simulink model "prob_8"  (R2020b)
settings: Solver=VariableStepAuto  StartTime=0.0  StopTime=10.0  RelTol=1e-3
settings Model: Creator=Akshay A H  LastModifiedBy=Akshay A H

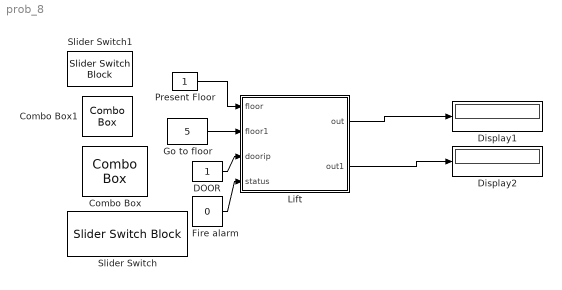
== system prob_8 ==
  Combo Box : ComboBox  SelectedLabel=FLOOR4
      settings: Values={{'GROUND', 'FLOOR1', 'FLOOR2', 'FLOOR3', 'FLOOR4'}, [1 2 3 4 5]}
  Combo Box1 : ComboBox  SelectedLabel=GROUND
      settings: Values={{'GROUND', 'FLOOR1', 'FLOOR2', 'FLOOR3', 'FLOOR4'}, [1 2 3 4 5]}
  DOOR : Constant
  Display1 : Display
  Display2 : Display
  Fire alarm : Constant  Value=0
  Go to floor : Constant  Value=5
  Lift : Stateflow chart  TreatAsAtomicUnit=on
  Present Floor : Constant
  Slider Switch : SliderSwitchBlock
      settings: Values={{'Off', 'On'}, [0 1]}
  Slider Switch1 : SliderSwitchBlock
      settings: Values={{'Off', 'On'}, [0 1]}
  wires:
  Present Floor/1 -> Lift/1(floor)
  Lift/1(out) -> Display1/1
  Lift/2(out1) -> Display2/1
  DOOR/1 -> Lift/3(doorip)
  Go to floor/1 -> Lift/2(floor1)
  Fire alarm/1 -> Lift/4(status)

== stateflow chart prob_8/Lift ==
  state Start
    (history)
    state Lift_For_five_floor
      (history)
      state Floor1
        entry:
        present=1;
        out=1;
      state Floor2
        entry:
        out=2;
        present=out;
      state Floor3
        entry:
        out=3;
        present=out;
      state Floor4
        entry:
        out=4;
        present=out;
      state Floor5
        entry:
        out=5;
        present=out
      Start.Lift_For_five_floor.Floor1 -> Start.Lift_For_five_floor.Floor1 [order 2] : [present==floor]
      (default) -> Start.Lift_For_five_floor.Floor1
      Start.Lift_For_five_floor.Floor3 -> Start.Lift_For_five_floor.Floor4 [order 1] : [present<floor]
      Start.Lift_For_five_floor.Floor2 -> Start.Lift_For_five_floor.Floor3 [order 1] : [present<floor]
      Start.Lift_For_five_floor.Floor4 -> Start.Lift_For_five_floor.Floor5 [order 1] : [present<floor]
      Start.Lift_For_five_floor.Floor1 -> Start.Lift_For_five_floor.Floor2 [order 1] : [present<floor]
      Start.Lift_For_five_floor.Floor5 -> Start.Lift_For_five_floor.Floor5 [order 2] : [floor==present]
      Start.Lift_For_five_floor.Floor5 -> Start.Lift_For_five_floor.Floor4 [order 1] : [present>floor]
      Start.Lift_For_five_floor.Floor4 -> Start.Lift_For_five_floor.Floor3 [order 2] : [present>floor]
      Start.Lift_For_five_floor.Floor2 -> Start.Lift_For_five_floor.Floor1 [order 2] : [present>floor]
      Start.Lift_For_five_floor.Floor3 -> Start.Lift_For_five_floor.Floor2 [order 2] : [present>floor]
    state Second_input
      (history)
      state Floor1
        entry:
        present=1
        if(status==1)
        out = floor1;
        end
        out1=1;
      state Floor2
        entry:
        out1=2;
        if(status==1)
        out = floor1;
        end
        present=out1;
      state Floor3
        entry:
        out1=3;
        if(status==1)
        out = floor1;
        end
        present=out1;
      state Floor4
        entry:
        out1=4;
        if(status==1)
        out = floor1;
        end
        present=out1;
      state Floor5
        entry:
        out1=5;
        if(status==1)
        out = floor1;
        end
        present=out1;
      Start.Second_input.Floor1 -> Start.Second_input.Floor1 [order 2] : [present==floor1]
      (default) -> Start.Second_input.Floor1
      Start.Second_input.Floor1 -> Start.Second_input.Floor2 [order 1] : [present<floor1]
      Start.Second_input.Floor3 -> Start.Second_input.Floor4 [order 1] : [present<floor1]
      Start.Second_input.Floor2 -> Start.Second_input.Floor3 [order 1] : [present<floor1]
      Start.Second_input.Floor4 -> Start.Second_input.Floor5 [order 1] : [present<floor1]
      Start.Second_input.Floor5 -> Start.Second_input.Floor5 [order 2] : [floor==present]
      Start.Second_input.Floor2 -> Start.Second_input.Floor1 [order 2] : [present>floor1]
      Start.Second_input.Floor5 -> Start.Second_input.Floor4 [order 1] : [present>floor1]
      Start.Second_input.Floor4 -> Start.Second_input.Floor3 [order 2] : [present>floor1]
      Start.Second_input.Floor3 -> Start.Second_input.Floor2 [order 2] : [present>floor1]
    (default) -> Lift_For_five_floor
    Lift_For_five_floor -> Second_input : [present==floor]
  state Door_off
    entry:
    out=floor;
    out1=0;
    (history)
  (default) -> Door_off
  Start -> Door_off : [doorip==0]
  Door_off -> Start : [doorip==1]
  data: floor input; present local; out output; floor1 input; out1 output; doorip input; status input
